simulink library "Telemaster_Lib"  (R2024b)
settings: Solver=VariableStepAuto  StartTime=0.0  StopTime=10.0  RelTol=1e-3
undefined symbols (not defined in the file): aircraft, alpha, beta, CD0, CL0, CLa, Clb, Clda, CLde, Cldr, Clp, CLq, Clr, CM0, CMa, CMde, CMq, Cnb, Cnda, Cndr, Cnp, Cnr, CYb, CYda, CYdr, CYp, CYr, dt, Earth, HM_ail, HM_ele, HM_rud, Hmalpha, Hmbeta, Hmele, Hmrud, motor, TO, WGS84
libraries: simulink_extras x21, simulink x4, aerolibtransform2 x2, shared6dof x1, aerolibatmos2 x1, aerolibasang x1, shared6dofsys x1
settings Model: Creator=igmso  LastModifiedBy=MASTER
settings RTWCC: GPUComputeCapability=3.5

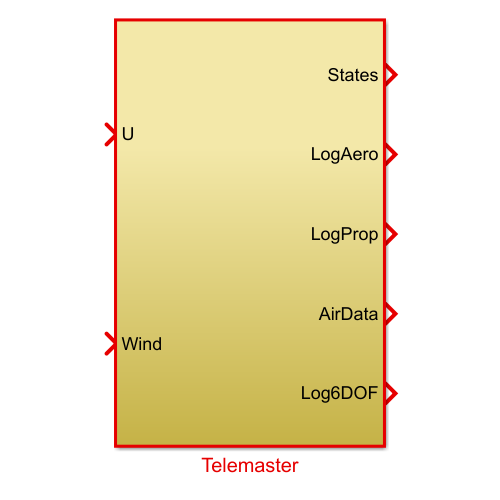
[thumbnail: Simulink's stored preview of the top-level diagram]
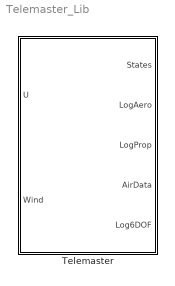
== system Telemaster_Lib ==
  Telemaster : Subsystem  TreatAsAtomicUnit=on

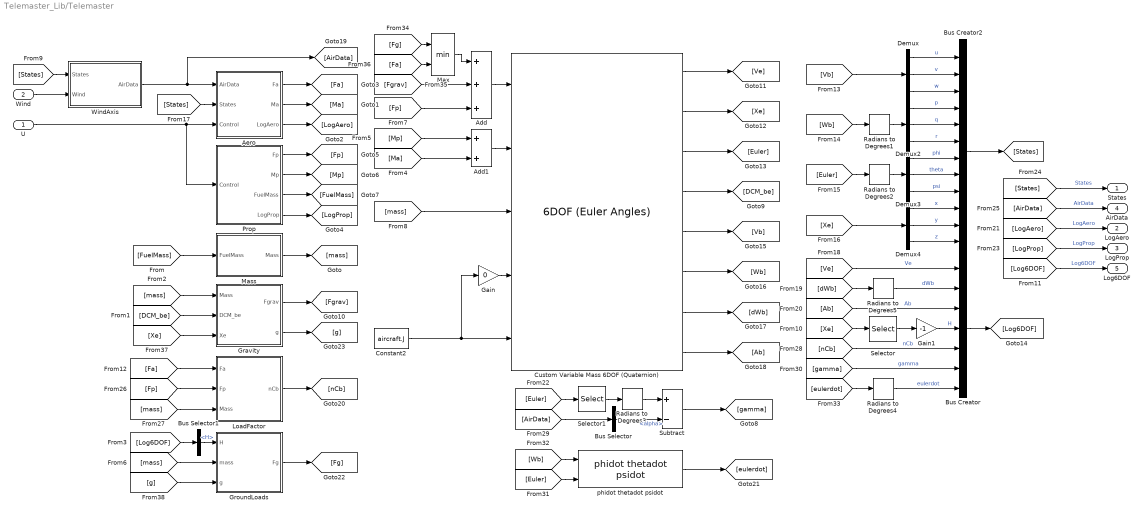
== system Telemaster_Lib/Telemaster ==
  U : Inport  SampleTime=dt
  Wind : Inport  Port=2  SampleTime=dt
  Add : Sum  Inputs=3
  Add1 : Sum
  Aero : Subsystem
  Bus Creator : BusCreator  Inputs=7
  Bus Creator2 : BusCreator  Inputs=12
  Bus Selector : BusSelector  OutputSignals=alpha
  Bus Selector1 : BusSelector  OutputSignals=H
  Constant2 : Constant  Value=aircraft.J  SampleTime=-1
  Custom Variable Mass 6DOF (Quaternion) : shared6dof/6DOF (Euler Angles)  units=Metric (MKS)  mtype=Custom Variable  rep=Euler Angles  xme_0=[TO.x TO.y TO.z-TO.alt0]  Vm_0=[TO.u TO.v TO.w]  eul_0=[TO.phi TO.theta TO.psi]  pm_0=[TO.p TO.q TO.r]  mass_0=1.0  mass_e=0.5  mass_f=2.0  inertia=eye(3)  inertia_e=eye(3)  inertia_f=2*eye(3)  k_quat=1.0  vre_flag=off  abi_flag=off  aMode=0  xme_statename={'Xe', 'Ye', 'Ze'}  Vm_statename={'u','v','w'}  eul_statename={'phi','theta','psi'}  quat_statename={'qr', 'qi', 'qj', 'qk'}  pm_statename={'p', 'q', 'r'}  mass_statename=''
  Demux{,2..4} (4 alike) : Demux  Outputs=3
  Gain : Gain  Gain=0
  Gain1 : Gain  Gain=-1
  Gravity : Subsystem
  GroundLoads : Subsystem
  LoadFactor : Subsystem
  Mass : Subsystem
  Max : MinMax  Inputs=2
  Prop : Subsystem
  Radians to Degrees{1..5} (5 alike) : simulink_extras/Transformations/Radians to Degrees
  Selector : Selector  InputPortWidth=3  IndexOptions=Index vector (dialog)  Indices=3  OutputSizes=1
  Selector1 : Selector  InputPortWidth=3  IndexOptions=Index vector (dialog)  Indices=2  OutputSizes=1
  Subtract : Sum  Inputs=+-
  WindAxis : Subsystem
  phidot thetadot psidot : shared6dofsys/DCM & Euler Angles (Euler)/phidot thetadot psidot  SystemSampleTime=-1  VariantActivationTime=update diagram  AllowFlexibleInterface=on  Latency=0  AutoFrameSizeCalculation=off
  States : Outport  SampleTime=dt
  LogAero : Outport  Port=2  SampleTime=dt
  LogProp : Outport  Port=3  SampleTime=dt
  AirData : Outport  Port=4  SampleTime=dt
  Log6DOF : Outport  Port=5  SampleTime=dt
  wires:
  [Ma] -> Add1/2
  [g] -> GroundLoads/3(g)
  Gravity/2(g) -> [g]
  [Xe] -> Gravity/3(Xe)
  [mass] -> GroundLoads/2(mass)
  Add1/1 -> Custom Variable Mass 6DOF (Quaternion)/2
  [Fa] -> Max/2
  [Fp] -> Add/3
  Max/1 -> Add/1
  [Fg] -> Max/1
  [Fgrav] -> Add/2
  Add/1 -> Custom Variable Mass 6DOF (Quaternion)/1
  [Mp] -> Add1/1
  GroundLoads/1(Fg) -> [Fg]
  Bus Selector1/1 -> GroundLoads/1(H)  "<H>"
  [Log6DOF] -> Bus Selector1/1
  Radians to Degrees5/1 -> Bus Creator/2  "dWb"
  Radians to Degrees4/1 -> Bus Creator/7  "eulerdot"
  [eulerdot] -> Radians to Degrees4/1
  phidot thetadot psidot/1 -> [eulerdot]
  [Wb] -> phidot thetadot psidot/1
  [Euler] -> phidot thetadot psidot/2
  Subtract/1 -> [gamma]
  Bus Selector/1 -> Subtract/2  "<alpha>"
  [AirData] -> Bus Selector/1
  Selector1/1 -> Radians to Degrees3/1
  Radians to Degrees3/1 -> Subtract/1
  [Euler] -> Selector1/1
  [gamma] -> Bus Creator/6  "gamma"
  [nCb] -> Bus Creator/5  "nCb"
  LoadFactor/1(nCb) -> [nCb]
  [mass] -> LoadFactor/3(Mass)
  [Fa] -> LoadFactor/1(Fa)
  [Fp] -> LoadFactor/2(Fp)
  [Log6DOF] -> Log6DOF/1  "Log6DOF"
  Bus Creator/1 -> [Log6DOF]
  Gain1/1 -> Bus Creator/4  "H"
  Selector/1 -> Gain1/1
  [Xe] -> Selector/1
  [Ab] -> Bus Creator/3  "Ab"
  [dWb] -> Radians to Degrees5/1
  [Ve] -> Bus Creator/1  "Ve"
  [States] -> States/1  "States"
  [LogProp] -> LogProp/1  "LogProp"
  [LogAero] -> LogAero/1  "LogAero"
  [AirData] -> AirData/1  "AirData"
  U/1 -> Aero/3(Control), Prop/1(Control)
  Demux3/3 -> Bus Creator2/9  "psi"
  Custom Variable Mass 6DOF (Quaternion)/4 -> [DCM_be]
  Demux3/1 -> Bus Creator2/7  "phi"
  Bus Creator2/1 -> [States]
  Custom Variable Mass 6DOF (Quaternion)/3 -> [Euler]
  Wind/1 -> WindAxis/2(Wind)
  [mass] -> Gravity/1(Mass)
  Demux4/2 -> Bus Creator2/11  "y"
  Custom Variable Mass 6DOF (Quaternion)/7 -> [dWb]
  Demux/3 -> Bus Creator2/3  "w"
  Aero/2(Ma) -> [Ma]
  Aero/1(Fa) -> [Fa]
  Custom Variable Mass 6DOF (Quaternion)/8 -> [Ab]
  [FuelMass] -> Mass/1(FuelMass)
  Demux3/2 -> Bus Creator2/8  "theta"
  Demux/2 -> Bus Creator2/2  "v"
  [States] -> Aero/2(States)
  [mass] -> Custom Variable Mass 6DOF (Quaternion)/3
  Custom Variable Mass 6DOF (Quaternion)/2 -> [Xe]
  [Vb] -> Demux/1
  Gain/1 -> Custom Variable Mass 6DOF (Quaternion)/4
  Gravity/1(Fgrav) -> [Fgrav]
  Constant2/1 -> Custom Variable Mass 6DOF (Quaternion)/5, Gain/1
  Radians to Degrees2/1 -> Demux3/1
  Mass/1(Mass) -> [mass]
  Prop/3(FuelMass) -> [FuelMass]
  Demux4/1 -> Bus Creator2/10  "x"
  Custom Variable Mass 6DOF (Quaternion)/1 -> [Ve]
  [Euler] -> Radians to Degrees2/1
  Demux2/2 -> Bus Creator2/5  "q"
  Prop/2(Mp) -> [Mp]
  Demux/1 -> Bus Creator2/1  "u"
  Prop/1(Fp) -> [Fp]
  [Wb] -> Radians to Degrees1/1
  Demux2/3 -> Bus Creator2/6  "r"
  Custom Variable Mass 6DOF (Quaternion)/6 -> [Wb]
  Demux4/3 -> Bus Creator2/12  "z"
  Custom Variable Mass 6DOF (Quaternion)/5 -> [Vb]
  [States] -> WindAxis/1(States)
  Demux2/1 -> Bus Creator2/4  "p"
  WindAxis/1(AirData) -> [AirData], Aero/1(AirData)
  Aero/3(LogAero) -> [LogAero]
  [DCM_be] -> Gravity/2(DCM_be)
  [Xe] -> Demux4/1
  Prop/4(LogProp) -> [LogProp]
  Radians to Degrees1/1 -> Demux2/1

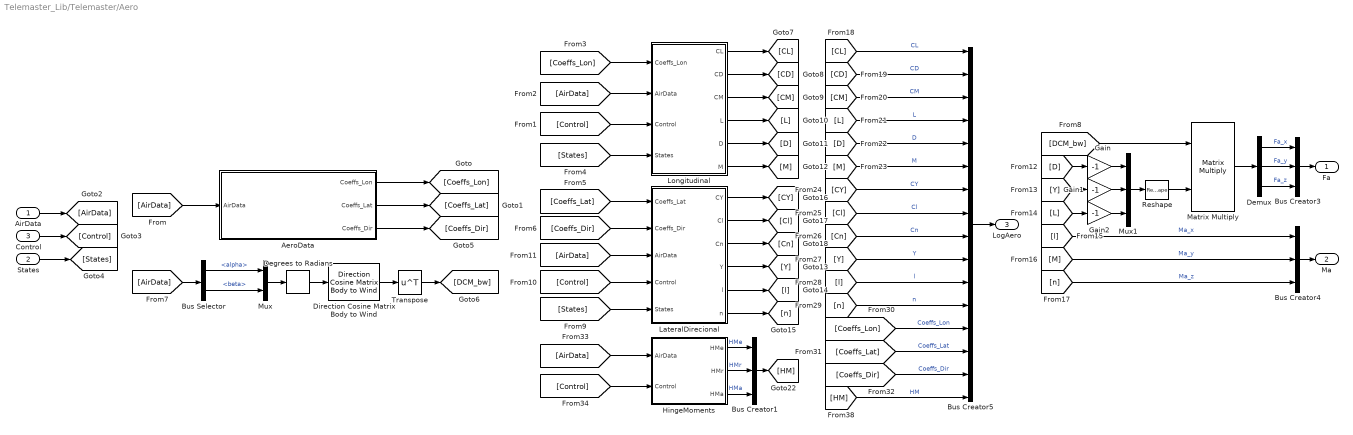
== system Telemaster_Lib/Telemaster/Aero ==
  AirData : Inport  SampleTime=dt
  States : Inport  Port=2  SampleTime=dt
  Control : Inport  Port=3  SampleTime=dt
  AeroData : Subsystem
  Bus Selector : BusSelector  OutputSignals=alpha,beta
  Bus Creator1 : BusCreator  Inputs=3
  Bus Creator3 : BusCreator  Inputs=3
  Bus Creator4 : BusCreator  Inputs=3
  Bus Creator5 : BusCreator  Inputs=16
  Degrees to Radians : simulink_extras/Transformations/Degrees to Radians
  Demux : Demux  Outputs=3
  Direction Cosine Matrix Body to Wind : aerolibtransform2/Direction Cosine Matrix Body to Wind
  Gain : Gain  Gain=-1
  Gain1 : Gain  Gain=-1
  Gain2 : Gain  Gain=-1
  HingeMoments : Subsystem
  LateralDirecional : Subsystem
  Longitudinal : Subsystem
  Matrix Multiply : Product  Multiplication=Matrix(*)
  Mux : Mux  Inputs=2
  Mux1 : Mux  Inputs=3
  Reshape : Reshape  OutputDimensionality=Column vector (2-D)
  Transpose : Math  Operator=transpose
  Fa : Outport  SampleTime=dt
  Ma : Outport  Port=2  SampleTime=dt
  LogAero : Outport  Port=3  SampleTime=dt
  wires:
  [HM] -> Bus Creator5/16  "HM"
  Reshape/1 -> Matrix Multiply/2
  Gain2/1 -> Mux1/3
  Gain1/1 -> Mux1/2
  Gain/1 -> Mux1/1
  Bus Selector/2 -> Mux/2  "<beta>"
  Bus Selector/1 -> Mux/1  "<alpha>"
  [AirData] -> Bus Selector/1
  [AirData] -> AeroData/1(AirData)
  AirData/1 -> [AirData]
  Bus Creator1/1 -> [HM]
  HingeMoments/1(HMe) -> Bus Creator1/1  "HMe"
  HingeMoments/2(HMr) -> Bus Creator1/2  "HMr"
  HingeMoments/3(HMa) -> Bus Creator1/3  "HMa"
  [Control] -> HingeMoments/2(Control)
  [AirData] -> HingeMoments/1(AirData)
  Control/1 -> [Control]
  Bus Creator4/1 -> Ma/1
  LateralDirecional/4(Y) -> [Y]
  [Coeffs_Dir] -> Bus Creator5/15  "Coeffs_Dir"
  LateralDirecional/1(CY) -> [CY]
  [L] -> Gain2/1
  Longitudinal/3(CM) -> [CM]
  [DCM_bw] -> Matrix Multiply/1
  Direction Cosine Matrix Body to Wind/1 -> Transpose/1
  [AirData] -> Longitudinal/2(AirData)
  States/1 -> [States]
  Mux1/1 -> Reshape/1
  Mux/1 -> Degrees to Radians/1
  AeroData/2(Coeffs_Lat) -> [Coeffs_Lat]
  AeroData/3(Coeffs_Dir) -> [Coeffs_Dir]
  [States] -> LateralDirecional/5(States)
  Bus Creator5/1 -> LogAero/1
  [Control] -> LateralDirecional/4(Control)
  [CL] -> Bus Creator5/1  "CL"
  Longitudinal/4(L) -> [L]
  [Coeffs_Lon] -> Bus Creator5/13  "Coeffs_Lon"
  [l] -> Bus Creator5/11  "l"
  [n] -> Bus Creator5/12  "n"
  [Cn] -> Bus Creator5/9  "Cn"
  Matrix Multiply/1 -> Demux/1
  [M] -> Bus Creator5/6  "M"
  [CM] -> Bus Creator5/3  "CM"
  Transpose/1 -> [DCM_bw]
  Longitudinal/2(CD) -> [CD]
  Bus Creator3/1 -> Fa/1
  [Coeffs_Dir] -> LateralDirecional/2(Coeffs_Dir)
  [CY] -> Bus Creator5/7  "CY"
  [M] -> Bus Creator4/2  "Ma_y"
  [D] -> Bus Creator5/5  "D"
  Longitudinal/1(CL) -> [CL]
  [L] -> Bus Creator5/4  "L"
  [l] -> Bus Creator4/1  "Ma_x"
  [Control] -> Longitudinal/3(Control)
  LateralDirecional/6(n) -> [n]
  Demux/3 -> Bus Creator3/3  "Fa_z"
  LateralDirecional/3(Cn) -> [Cn]
  LateralDirecional/5(l) -> [l]
  [Coeffs_Lat] -> LateralDirecional/1(Coeffs_Lat)
  [States] -> Longitudinal/4(States)
  Degrees to Radians/1 -> Direction Cosine Matrix Body to Wind/1
  [Y] -> Gain1/1
  Demux/1 -> Bus Creator3/1  "Fa_x"
  AeroData/1(Coeffs_Lon) -> [Coeffs_Lon]
  Demux/2 -> Bus Creator3/2  "Fa_y"
  LateralDirecional/2(Cl) -> [Cl]
  [D] -> Gain/1
  Longitudinal/5(D) -> [D]
  [Cl] -> Bus Creator5/8  "Cl"
  [Coeffs_Lat] -> Bus Creator5/14  "Coeffs_Lat"
  [n] -> Bus Creator4/3  "Ma_z"
  Longitudinal/6(M) -> [M]
  [CD] -> Bus Creator5/2  "CD"
  [Y] -> Bus Creator5/10  "Y"
  [Coeffs_Lon] -> Longitudinal/1(Coeffs_Lon)
  [AirData] -> LateralDirecional/3(AirData)

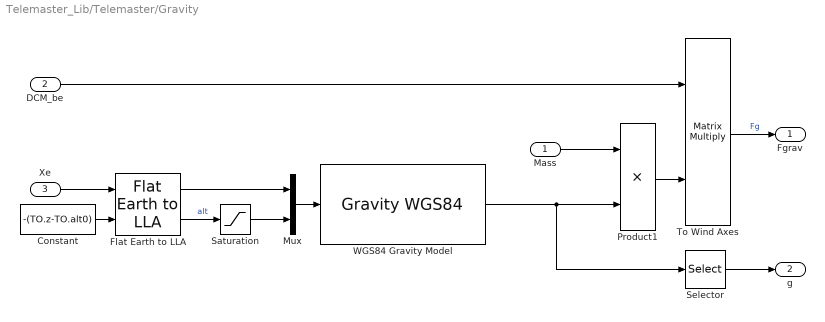
== system Telemaster_Lib/Telemaster/Gravity ==
  Mass : Inport  SampleTime=dt
  DCM_be : Inport  Port=2  SampleTime=dt
  Xe : Inport  Port=3
  Constant : Constant  Value=-(TO.z-TO.alt0)  SampleTime=-1
  Flat Earth to LLA : aerolibtransform2/Flat Earth to LLA  units=Metric (MKS)  ptype=Earth (WGS84)  F=1/298.257223563  R=6378137  refPosPort=off  LL0=[-23.2296 -45.8614].'  psi=150
  Mux : Mux  Inputs=2
  Product1 : Product
  Saturation : Saturate  UpperLimit=20e3  LowerLimit=0
  Selector : Selector  InputPortWidth=3  IndexOptions=Index vector (dialog)  Indices=3  OutputSizes=1
  To Wind Axes : Product  Multiplication=Matrix(*)  InputSameDT=on  SaturateOnIntegerOverflow=on  OutDataTypeStr=Inherit: Same as first input
  "WGS84 Gravity Model  " : GravityWGS84
  Fgrav : Outport  SampleTime=dt
  g : Outport  Port=2
  wires:
  Selector/1 -> g/1
  Mass/1 -> Product1/1
  Saturation/1 -> Mux/2
  Xe/1 -> Flat Earth to LLA/1
  "WGS84 Gravity Model  "/1 -> Product1/2, Selector/1
  Flat Earth to LLA/1 -> Mux/1
  DCM_be/1 -> To Wind Axes/1
  To Wind Axes/1 -> Fgrav/1  "Fg"
  Product1/1 -> To Wind Axes/2
  Mux/1 -> "WGS84 Gravity Model  "/1
  Flat Earth to LLA/2 -> Saturation/1  "alt"
  Constant/1 -> Flat Earth to LLA/2

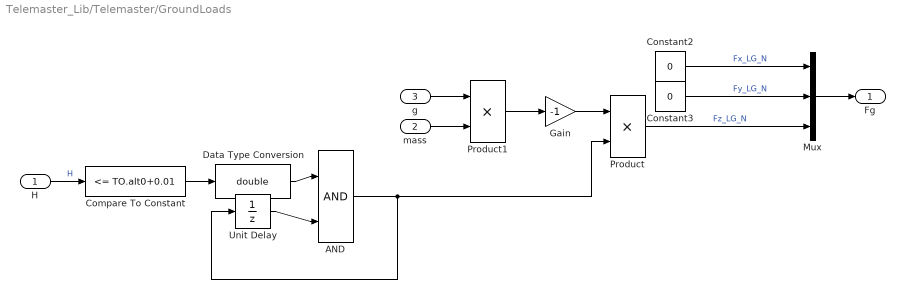
== system Telemaster_Lib/Telemaster/GroundLoads ==
  H : Inport
  mass : Inport  Port=2
  g : Inport  Port=3
  AND : Logic  IconShape=distinctive  AllPortsSameDT=off  OutDataTypeStr=boolean
  Compare To Constant : simulink/Logic and Bit Operations/Compare To Constant  relop=<=  const=TO.alt0+0.01  OutDataTypeStr=boolean
  Constant2 : Constant  Value=0  SampleTime=-1
  Constant3 : Constant  Value=0  SampleTime=-1
  Data Type Conversion : DataTypeConversion  OutDataTypeStr=double  SaturateOnIntegerOverflow=off  RndMeth=Floor
  Gain : Gain  Gain=-1
  Mux : Mux  Inputs=3
  Product : Product
  Product1 : Product
  Unit Delay : UnitDelay  InitialCondition=1  SampleTime=-1  HasFrameUpgradeWarning=on
  Fg : Outport
  wires:
  AND/1 -> Unit Delay/1, Product/2
  Gain/1 -> Product/1
  g/1 -> Product1/1
  Mux/1 -> Fg/1
  Product/1 -> Mux/3  "Fz_LG_N"
  Constant3/1 -> Mux/2  "Fy_LG_N"
  Constant2/1 -> Mux/1  "Fx_LG_N"
  H/1 -> Compare To Constant/1  "H"
  Compare To Constant/1 -> Data Type Conversion/1
  Product1/1 -> Gain/1
  mass/1 -> Product1/2
  Data Type Conversion/1 -> AND/1
  Unit Delay/1 -> AND/2

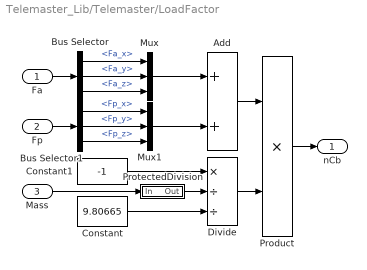
== system Telemaster_Lib/Telemaster/LoadFactor ==
  Fa : Inport  SampleTime=dt
  Fp : Inport  Port=2  SampleTime=dt
  Mass : Inport  Port=3  SampleTime=dt
  Add : Sum  Inputs=2
  Bus Selector : BusSelector  OutputSignals=Fa_x,Fa_y,Fa_z
  Bus Selector1 : BusSelector  OutputSignals=Fp_x,Fp_y,Fp_z
  Constant : Constant  Value=9.80665  SampleTime=dt
  Constant1 : Constant  Value=-1  SampleTime=dt
  Divide : Product  Inputs=*//
  Mux : Mux  Inputs=3
  Mux1 : Mux  Inputs=3
  Product : Product
  ProtectedDivision : Subsystem
  nCb : Outport  SampleTime=dt
  wires:
  ProtectedDivision/1(Out) -> Divide/2
  Product/1 -> nCb/1
  Divide/1 -> Product/2
  Constant/1 -> Divide/3
  Mass/1 -> ProtectedDivision/1(In)
  Constant1/1 -> Divide/1
  Add/1 -> Product/1
  Fa/1 -> Bus Selector/1
  Bus Selector/1 -> Mux/1  "<Fa_x>"
  Bus Selector/2 -> Mux/2  "<Fa_y>"
  Bus Selector/3 -> Mux/3  "<Fa_z>"
  Fp/1 -> Bus Selector1/1
  Bus Selector1/1 -> Mux1/1  "<Fp_x>"
  Bus Selector1/2 -> Mux1/2  "<Fp_y>"
  Bus Selector1/3 -> Mux1/3  "<Fp_z>"
  Mux/1 -> Add/1
  Mux1/1 -> Add/2

== system Telemaster_Lib/Telemaster/Mass ==
  FuelMass : Inport  SampleTime=dt
  Add : Sum
  Constant1 : Constant  Value=aircraft.m  SampleTime=dt
  Mass : Outport  SampleTime=dt
  wires:
  Add/1 -> Mass/1
  FuelMass/1 -> Add/2
  Constant1/1 -> Add/1

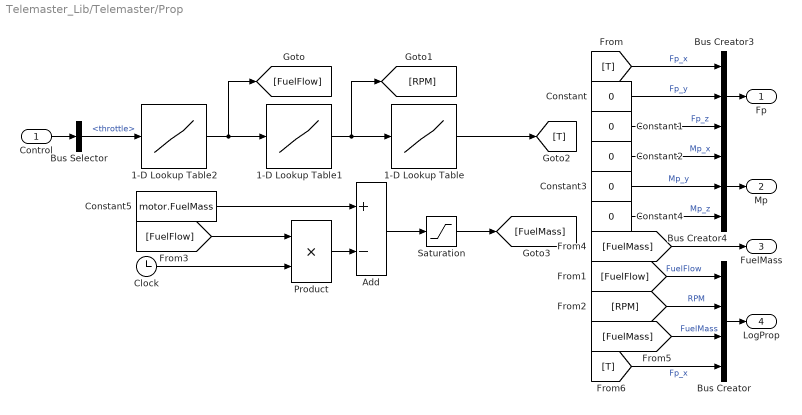
== system Telemaster_Lib/Telemaster/Prop ==
  Control : Inport  SampleTime=dt
  1-D Lookup Table : Lookup_n-D  NumberOfTableDimensions=1  BreakpointsForDimension1=[1600 6600]  Table=[0 28.4]  ExtrapMethod=Clip  InternalRulePriority=Speed  RndMeth=Simplest
  1-D Lookup Table1 : Lookup_n-D  NumberOfTableDimensions=1  BreakpointsForDimension1=[0.0002 0.001]  Table=[1600 6600]  ExtrapMethod=Clip  InternalRulePriority=Speed  RndMeth=Simplest
  1-D Lookup Table2 : Lookup_n-D  NumberOfTableDimensions=1  BreakpointsForDimension1=[0 1]  Table=[0.0002 0.001]  ExtrapMethod=Clip  InternalRulePriority=Speed  RndMeth=Simplest
  Add : Sum  Inputs=+-
  Bus Selector : BusSelector  OutputSignals=throttle
  Bus Creator : BusCreator  Inputs=4
  Bus Creator3 : BusCreator  Inputs=3
  Bus Creator4 : BusCreator  Inputs=3
  Clock : Clock
  Constant{,1..4} (5 alike) : Constant  Value=0  SampleTime=-1
  Constant5 : Constant  Value=motor.FuelMass  SampleTime=-1
  Product : Product
  Saturation : Saturate  UpperLimit=inf  LowerLimit=0
  Fp : Outport  SampleTime=dt
  Mp : Outport  Port=2  SampleTime=dt
  FuelMass : Outport  Port=3  SampleTime=dt
  LogProp : Outport  Port=4  SampleTime=dt
  wires:
  [T] -> Bus Creator/4  "Fp_x"
  Clock/1 -> Product/2
  1-D Lookup Table2/1 -> 1-D Lookup Table1/1, [FuelFlow]
  1-D Lookup Table1/1 -> 1-D Lookup Table/1, [RPM]
  1-D Lookup Table/1 -> [T]
  Bus Selector/1 -> 1-D Lookup Table2/1  "<throttle>"
  [FuelMass] -> Bus Creator/3  "FuelMass"
  [FuelFlow] -> Bus Creator/1  "FuelFlow"
  Saturation/1 -> [FuelMass]
  Bus Creator/1 -> LogProp/1
  [RPM] -> Bus Creator/2  "RPM"
  [FuelMass] -> FuelMass/1
  Add/1 -> Saturation/1
  Product/1 -> Add/2
  [FuelFlow] -> Product/1
  Constant5/1 -> Add/1
  Constant2/1 -> Bus Creator4/1  "Mp_x"
  Constant3/1 -> Bus Creator4/2  "Mp_y"
  [T] -> Bus Creator3/1  "Fp_x"
  Control/1 -> Bus Selector/1
  Constant/1 -> Bus Creator3/2  "Fp_y"
  Constant1/1 -> Bus Creator3/3  "Fp_z"
  Bus Creator3/1 -> Fp/1
  Bus Creator4/1 -> Mp/1
  Constant4/1 -> Bus Creator4/3  "Mp_z"

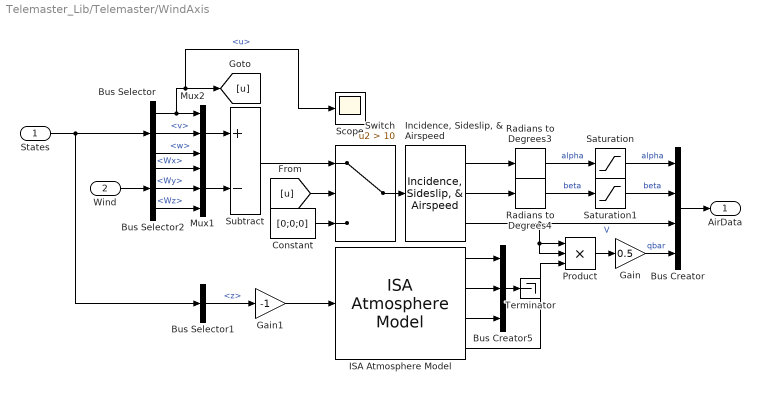
== system Telemaster_Lib/Telemaster/WindAxis ==
  States : Inport  SampleTime=dt
  Wind : Inport  Port=2  SampleTime=dt
  Bus Selector : BusSelector  OutputSignals=u,v,w
  Bus Selector1 : BusSelector  OutputSignals=z
  Bus Selector2 : BusSelector  OutputSignals=Wx,Wy,Wz
  Bus Creator : BusCreator  Inputs=4
  Bus Creator5 : BusCreator  Inputs=3
  Constant : Constant  Value=[0;0;0]  SampleTime=-1
  Gain : Gain  Gain=0.5
  Gain1 : Gain  Gain=-1
  ISA Atmosphere Model : aerolibatmos2/ISA Atmosphere Model  useExtended=off  action=Warning  custom=off  viscosityOut=off  g=9.80665  gamma=1.4  R=287.0531  L=0.0065  h_trop=11000  h_strat=20000  rho0=1.225  P0=101325  T0=288.15  h0=0  S=110.4  Tref=273.15  muref=1.716e-5
  "Incidence, Sideslip, & Airspeed" : aerolibasang/Incidence, Sideslip, & Airspeed
  Mux1 : Mux  Inputs=3
  Mux2 : Mux  Inputs=3
  Product : Product  Inputs=3
  Radians to Degrees3 : simulink_extras/Transformations/Radians to Degrees
  Radians to Degrees4 : simulink_extras/Transformations/Radians to Degrees
  Saturation : Saturate  UpperLimit=15  LowerLimit=-10
  Saturation1 : Saturate  UpperLimit=10  LowerLimit=-10
  Scope : Scope
  Subtract : Sum  Inputs=+-
  Switch : Switch  Criteria=u2 > Threshold  Threshold=10  SaturateOnIntegerOverflow=off  InputSameDT=off
  Terminator : Terminator
  AirData : Outport  SampleTime=dt
  wires:
  Constant/1 -> Switch/3
  Switch/1 -> "Incidence, Sideslip, & Airspeed"/1
  [u] -> Switch/2
  Saturation1/1 -> Bus Creator/2  "beta"
  Saturation/1 -> Bus Creator/1  "alpha"
  Mux2/1 -> Subtract/1
  Product/1 -> Gain/1
  Wind/1 -> Bus Selector2/1
  Bus Selector2/3 -> Mux1/3  "<Wz>"
  Bus Selector2/1 -> Mux1/1  "<Wx>"
  Mux1/1 -> Subtract/2
  Bus Selector2/2 -> Mux1/2  "<Wy>"
  Bus Creator/1 -> AirData/1
  "Incidence, Sideslip, & Airspeed"/1 -> Radians to Degrees3/1
  ISA Atmosphere Model/2 -> Bus Creator5/2
  ISA Atmosphere Model/1 -> Bus Creator5/1
  Radians to Degrees4/1 -> Saturation1/1  "beta"
  Gain/1 -> Bus Creator/4  "qbar"
  Bus Selector/2 -> Mux2/2  "<v>"
  ISA Atmosphere Model/4 -> Product/3
  ISA Atmosphere Model/3 -> Bus Creator5/3
  Bus Selector/1 -> Mux2/1, [u], Scope/1  "<u>"
  Radians to Degrees3/1 -> Saturation/1  "alpha"
  Bus Selector1/1 -> Gain1/1  "<z>"
  Gain1/1 -> ISA Atmosphere Model/1
  "Incidence, Sideslip, & Airspeed"/3 -> Product/1, Product/2, Bus Creator/3  "V"
  States/1 -> Bus Selector/1, Bus Selector1/1
  Bus Creator5/1 -> Terminator/1
  "Incidence, Sideslip, & Airspeed"/2 -> Radians to Degrees4/1
  Subtract/1 -> Switch/1
  Bus Selector/3 -> Mux2/3  "<w>"

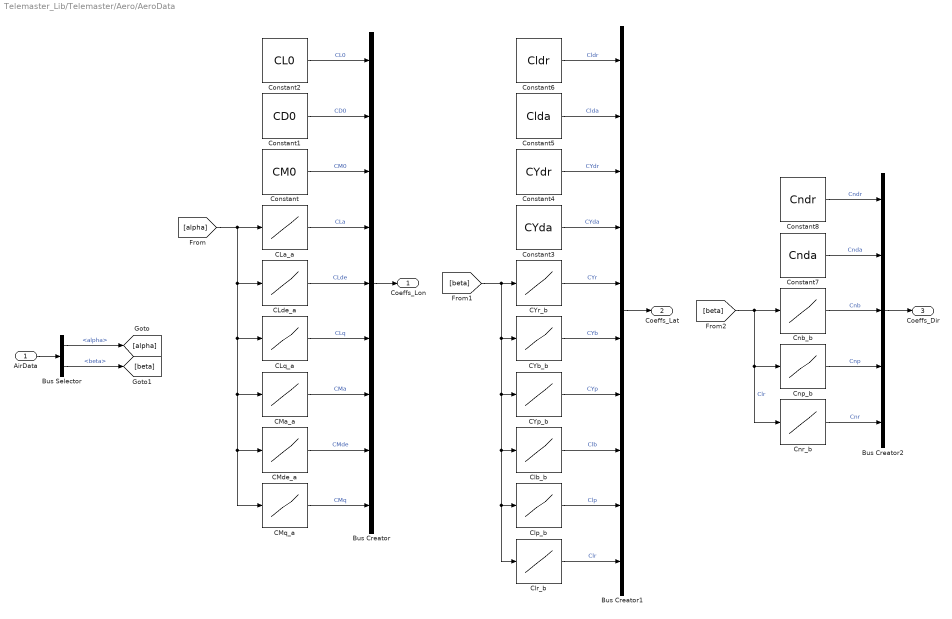
== system Telemaster_Lib/Telemaster/Aero/AeroData ==
  AirData : Inport
  Bus Selector : BusSelector  OutputSignals=alpha,beta
  Bus Creator : BusCreator  Inputs=9
  Bus Creator1 : BusCreator  Inputs=10
  Bus Creator2 : BusCreator  Inputs=5
  CLa_a : Lookup_n-D  NumberOfTableDimensions=1  BreakpointsForDimension1=alpha  Table=CLa  InternalRulePriority=Speed  RndMeth=Simplest
  CLde_a : Lookup_n-D  NumberOfTableDimensions=1  BreakpointsForDimension1=alpha  Table=CLde  InternalRulePriority=Speed  RndMeth=Simplest
  CLq_a : Lookup_n-D  NumberOfTableDimensions=1  BreakpointsForDimension1=alpha  Table=CLq  InternalRulePriority=Speed  RndMeth=Simplest
  CMa_a : Lookup_n-D  NumberOfTableDimensions=1  BreakpointsForDimension1=alpha  Table=CMa  InternalRulePriority=Speed  RndMeth=Simplest
  CMde_a : Lookup_n-D  NumberOfTableDimensions=1  BreakpointsForDimension1=alpha  Table=CMde  InternalRulePriority=Speed  RndMeth=Simplest
  CMq_a : Lookup_n-D  NumberOfTableDimensions=1  BreakpointsForDimension1=alpha  Table=CMq  InternalRulePriority=Speed  RndMeth=Simplest
  CYb_b : Lookup_n-D  NumberOfTableDimensions=1  BreakpointsForDimension1=beta  Table=CYb  InternalRulePriority=Speed  RndMeth=Simplest
  CYp_b : Lookup_n-D  NumberOfTableDimensions=1  BreakpointsForDimension1=beta  Table=CYp  InternalRulePriority=Speed  RndMeth=Simplest
  CYr_b : Lookup_n-D  NumberOfTableDimensions=1  BreakpointsForDimension1=beta  Table=CYr  InternalRulePriority=Speed  RndMeth=Simplest
  Clb_b : Lookup_n-D  NumberOfTableDimensions=1  BreakpointsForDimension1=beta  Table=Clb  InternalRulePriority=Speed  RndMeth=Simplest
  Clp_b : Lookup_n-D  NumberOfTableDimensions=1  BreakpointsForDimension1=beta  Table=Clp  InternalRulePriority=Speed  RndMeth=Simplest
  Clr_b : Lookup_n-D  NumberOfTableDimensions=1  BreakpointsForDimension1=beta  Table=Clr  InternalRulePriority=Speed  RndMeth=Simplest
  Cnb_b : Lookup_n-D  NumberOfTableDimensions=1  BreakpointsForDimension1=beta  Table=Cnb  InternalRulePriority=Speed  RndMeth=Simplest
  Cnp_b : Lookup_n-D  NumberOfTableDimensions=1  BreakpointsForDimension1=beta  Table=Cnp  InternalRulePriority=Speed  RndMeth=Simplest
  Cnr_b : Lookup_n-D  NumberOfTableDimensions=1  BreakpointsForDimension1=beta  Table=Cnr  InternalRulePriority=Speed  RndMeth=Simplest
  Constant : Constant  Value=CM0  SampleTime=-1
  Constant1 : Constant  Value=CD0  SampleTime=-1
  Constant2 : Constant  Value=CL0  SampleTime=-1
  Constant3 : Constant  Value=CYda  SampleTime=-1
  Constant4 : Constant  Value=CYdr  SampleTime=-1
  Constant5 : Constant  Value=Clda  SampleTime=-1
  Constant6 : Constant  Value=Cldr  SampleTime=-1
  Constant7 : Constant  Value=Cnda  SampleTime=-1
  Constant8 : Constant  Value=Cndr  SampleTime=-1
  Coeffs_Lon : Outport
  Coeffs_Lat : Outport  Port=2
  Coeffs_Dir : Outport  Port=3
  wires:
  Bus Selector/2 -> [beta]  "<beta>"
  Bus Selector/1 -> [alpha]  "<alpha>"
  AirData/1 -> Bus Selector/1
  Clr_b/1 -> Bus Creator1/10  "Clr"
  CYr_b/1 -> Bus Creator1/5  "CYr"
  Bus Creator2/1 -> Coeffs_Dir/1
  Cnp_b/1 -> Bus Creator2/4  "Cnp"
  Cnr_b/1 -> Bus Creator2/5  "Cnr"
  Cnb_b/1 -> Bus Creator2/3  "Cnb"
  [beta] -> Cnb_b/1, Cnp_b/1, Cnr_b/1  "Clr"
  Constant7/1 -> Bus Creator2/2  "Cnda"
  Constant8/1 -> Bus Creator2/1  "Cndr"
  Constant6/1 -> Bus Creator1/1  "Cldr"
  Constant5/1 -> Bus Creator1/2  "Clda"
  Constant4/1 -> Bus Creator1/3  "CYdr"
  Constant3/1 -> Bus Creator1/4  "CYda"
  Constant2/1 -> Bus Creator/1  "CL0"
  Constant1/1 -> Bus Creator/2  "CD0"
  Constant/1 -> Bus Creator/3  "CM0"
  Bus Creator1/1 -> Coeffs_Lat/1
  Bus Creator/1 -> Coeffs_Lon/1
  CLa_a/1 -> Bus Creator/4  "CLa"
  CMa_a/1 -> Bus Creator/7  "CMa"
  Clp_b/1 -> Bus Creator1/9  "Clp"
  CLde_a/1 -> Bus Creator/5  "CLde"
  CYb_b/1 -> Bus Creator1/6  "CYb"
  CMq_a/1 -> Bus Creator/9  "CMq"
  CLq_a/1 -> Bus Creator/6  "CLq"
  CYp_b/1 -> Bus Creator1/7  "CYp"
  Clb_b/1 -> Bus Creator1/8  "Clb"
  [beta] -> CYb_b/1, CYp_b/1, Clb_b/1, Clp_b/1, Clr_b/1, CYr_b/1
  CMde_a/1 -> Bus Creator/8  "CMde"
  [alpha] -> CLa_a/1, CLde_a/1, CLq_a/1, CMa_a/1, CMde_a/1, CMq_a/1

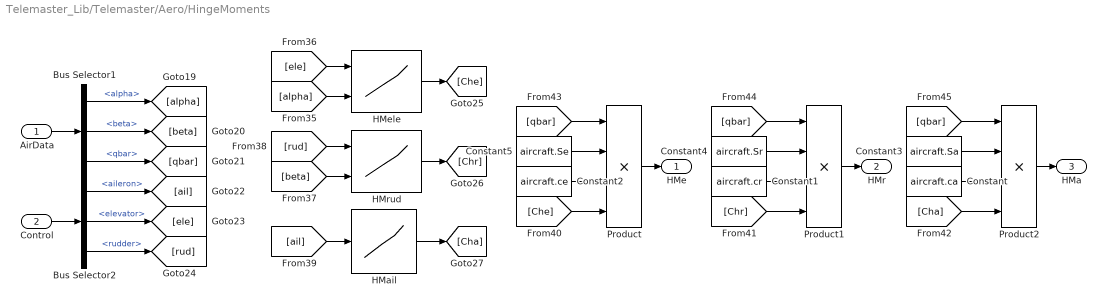
== system Telemaster_Lib/Telemaster/Aero/HingeMoments ==
  AirData : Inport
  Control : Inport  Port=2
  Bus Selector1 : BusSelector  OutputSignals=alpha,beta,qbar
  Bus Selector2 : BusSelector  OutputSignals=aileron,elevator,rudder
  Constant : Constant  Value=aircraft.ca  SampleTime=-1
  Constant1 : Constant  Value=aircraft.cr  SampleTime=-1
  Constant2 : Constant  Value=aircraft.ce  SampleTime=-1
  Constant3 : Constant  Value=aircraft.Sa  SampleTime=-1
  Constant4 : Constant  Value=aircraft.Sr  SampleTime=-1
  Constant5 : Constant  Value=aircraft.Se  SampleTime=-1
  HMail : Lookup_n-D  NumberOfTableDimensions=1  BreakpointsForDimension1=Hmrud  Table=HM_ail  InternalRulePriority=Speed  RndMeth=Simplest
  HMele : Lookup_n-D  BreakpointsForDimension1=Hmele  BreakpointsForDimension2=Hmalpha  Table=HM_ele  InternalRulePriority=Speed  RndMeth=Simplest
      settings: InputPortMap=u0,u1
  HMrud : Lookup_n-D  BreakpointsForDimension1=Hmrud  BreakpointsForDimension2=Hmbeta  Table=HM_rud  InternalRulePriority=Speed  RndMeth=Simplest
      settings: InputPortMap=u0,u1
  Product : Product  Inputs=4
  Product1 : Product  Inputs=4
  Product2 : Product  Inputs=4
  HMe : Outport
  HMr : Outport  Port=2
  HMa : Outport  Port=3
  wires:
  Product1/1 -> HMr/1
  Control/1 -> Bus Selector2/1
  AirData/1 -> Bus Selector1/1
  Bus Selector2/3 -> [rud]  "<rudder>"
  Bus Selector2/1 -> [ail]  "<aileron>"
  Constant4/1 -> Product1/2
  HMele/1 -> [Che]
  [rud] -> HMrud/1
  HMrud/1 -> [Chr]
  [ele] -> HMele/1
  [qbar] -> Product/1
  Bus Selector1/3 -> [qbar]  "<qbar>"
  Constant5/1 -> Product/2
  Constant2/1 -> Product/3
  Constant1/1 -> Product1/3
  [Chr] -> Product1/4
  Product2/1 -> HMa/1
  [Che] -> Product/4
  [beta] -> HMrud/2
  [qbar] -> Product1/1
  Bus Selector1/1 -> [alpha]  "<alpha>"
  Product/1 -> HMe/1
  [alpha] -> HMele/2
  Constant/1 -> Product2/3
  [qbar] -> Product2/1
  [Cha] -> Product2/4
  [ail] -> HMail/1
  Bus Selector1/2 -> [beta]  "<beta>"
  Constant3/1 -> Product2/2
  Bus Selector2/2 -> [ele]  "<elevator>"
  HMail/1 -> [Cha]

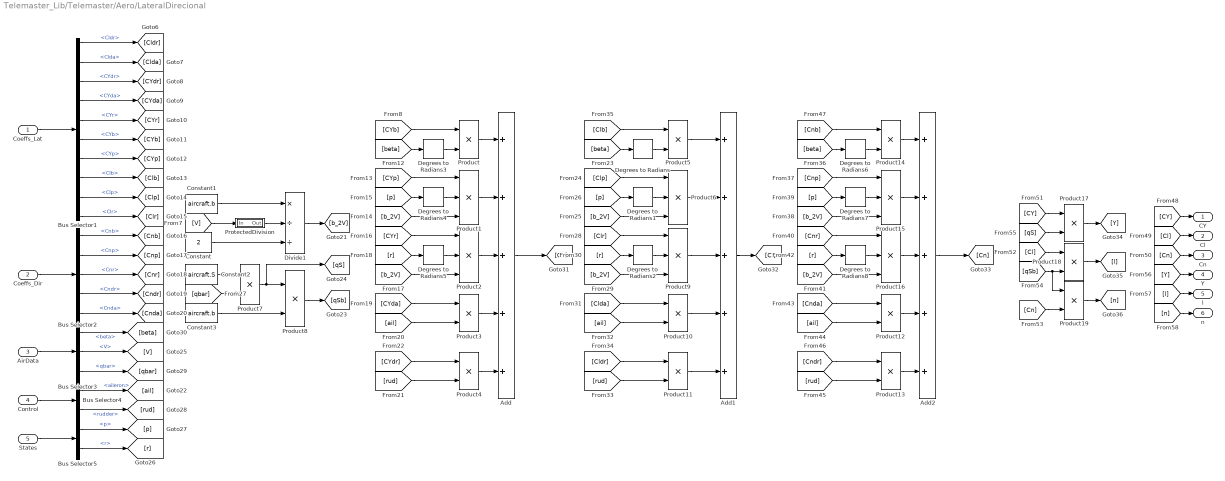
== system Telemaster_Lib/Telemaster/Aero/LateralDirecional ==
  Coeffs_Lat : Inport
  Coeffs_Dir : Inport  Port=2
  AirData : Inport  Port=3
  Control : Inport  Port=4
  States : Inport  Port=5
  Add : Sum  Inputs=5
  Add1 : Sum  Inputs=5
  Add2 : Sum  Inputs=5
  Bus Selector1 : BusSelector  OutputSignals=Cldr,Clda,CYdr,CYda,CYr,CYb,CYp,Clb,Clp,Clr
  Bus Selector2 : BusSelector  OutputSignals=Cnb,Cnp,Cnr,Cndr,Cnda
  Bus Selector3 : BusSelector  OutputSignals=beta,V,qbar
  Bus Selector4 : BusSelector  OutputSignals=aileron,rudder
  Bus Selector5 : BusSelector  OutputSignals=p,r
  Constant : Constant  Value=2  SampleTime=-1
  Constant1 : Constant  Value=aircraft.b  SampleTime=-1
  Constant2 : Constant  Value=aircraft.S
  Constant3 : Constant  Value=aircraft.b
  Degrees to Radians{,1..8} (9 alike) : simulink_extras/Transformations/Degrees to Radians
  Divide1 : Product  Inputs=*//
  Product{,3..5,7..8,10..14,17..19} (14 alike) : Product
  Product{1..2,6,9,15..16} (6 alike) : Product  Inputs=3
  ProtectedDivision : Subsystem
  CY : Outport
  Cl : Outport  Port=2
  Cn : Outport  Port=3
  Y : Outport  Port=4
  l : Outport  Port=5
  n : Outport  Port=6
  wires:
  ProtectedDivision/1(Out) -> Divide1/2
  [n] -> n/1
  Coeffs_Dir/1 -> Bus Selector2/1
  [Cl] -> Cl/1
  [CY] -> CY/1
  [l] -> l/1
  Control/1 -> Bus Selector4/1
  States/1 -> Bus Selector5/1
  Coeffs_Lat/1 -> Bus Selector1/1
  AirData/1 -> Bus Selector3/1
  Degrees to Radians/1 -> Product5/2
  Degrees to Radians2/1 -> Product9/2
  Product17/1 -> [Y]
  Add/1 -> [CY]
  [CYb] -> Product/1
  Bus Selector1/10 -> [Clr]  "<Clr>"
  [Clp] -> Product6/1
  [p] -> Degrees to Radians1/1
  [b_2V] -> Product6/3
  [Clb] -> Product5/1
  [Clda] -> Product10/1
  Product9/1 -> Add1/3
  Product5/1 -> Add1/1
  [ail] -> Product10/2
  [Clr] -> Product9/1
  Product10/1 -> Add1/4
  [r] -> Degrees to Radians2/1
  [b_2V] -> Product9/3
  Product6/1 -> Add1/2
  Add1/1 -> [Cl]
  Bus Selector2/4 -> [Cndr]  "<Cndr>"
  Bus Selector2/3 -> [Cnr]  "<Cnr>"
  Bus Selector5/1 -> [p]  "<p>"
  Degrees to Radians3/1 -> Product/2
  Bus Selector3/2 -> [V]  "<V>"
  Bus Selector4/1 -> [ail]  "<aileron>"
  Bus Selector4/2 -> [rud]  "<rudder>"
  Product19/1 -> [n]
  [p] -> Degrees to Radians4/1
  [r] -> Degrees to Radians5/1
  [b_2V] -> Product2/3
  Degrees to Radians8/1 -> Product16/2
  [CYda] -> Product3/1
  [CYdr] -> Product4/1
  Bus Selector2/1 -> [Cnb]  "<Cnb>"
  [Cldr] -> Product11/1
  [beta] -> Degrees to Radians3/1
  Bus Selector1/8 -> [Clb]  "<Clb>"
  [rud] -> Product11/2
  Degrees to Radians5/1 -> Product2/2
  Product/1 -> Add/1
  Product2/1 -> Add/3
  Divide1/1 -> [b_2V]
  [Cn] -> Product19/2
  [qbar] -> Product7/2
  [rud] -> Product4/2
  [Cl] -> Product18/1
  Degrees to Radians7/1 -> Product15/2
  Bus Selector5/2 -> [r]  "<r>"
  Product14/1 -> Add2/1
  [V] -> ProtectedDivision/1(In)
  [Cnb] -> Product14/1
  [b_2V] -> Product1/3
  Product11/1 -> Add1/5
  [ail] -> Product3/2
  Bus Selector1/9 -> [Clp]  "<Clp>"
  Bus Selector3/1 -> [beta]  "<beta>"
  Constant3/1 -> Product8/2
  Bus Selector1/7 -> [CYp]  "<CYp>"
  [Cn] -> Cn/1
  Product13/1 -> Add2/5
  [rud] -> Product13/2
  Bus Selector1/5 -> [CYr]  "<CYr>"
  [Cndr] -> Product13/1
  [qSb] -> Product18/2, Product19/1
  Bus Selector2/2 -> [Cnp]  "<Cnp>"
  Product3/1 -> Add/4
  Product15/1 -> Add2/2
  [Y] -> Y/1
  Bus Selector3/3 -> [qbar]  "<qbar>"
  [CYp] -> Product1/1
  Product16/1 -> Add2/3
  [ail] -> Product12/2
  Bus Selector2/5 -> [Cnda]  "<Cnda>"
  Bus Selector1/2 -> [Clda]  "<Clda>"
  Product7/1 -> Product8/1, [qS]
  Degrees to Radians4/1 -> Product1/2
  [Cnr] -> Product16/1
  [CYr] -> Product2/1
  [p] -> Degrees to Radians7/1
  Degrees to Radians6/1 -> Product14/2
  Bus Selector1/4 -> [CYda]  "<CYda>"
  Add2/1 -> [Cn]
  [r] -> Degrees to Radians8/1
  Bus Selector1/3 -> [CYdr]  "<CYdr>"
  Bus Selector1/1 -> [Cldr]  "<Cldr>"
  [b_2V] -> Product16/3
  [Cnda] -> Product12/1
  [qS] -> Product17/2
  [Cnp] -> Product15/1
  Product4/1 -> Add/5
  Constant/1 -> Divide1/3
  [CY] -> Product17/1
  Constant2/1 -> Product7/1
  [b_2V] -> Product15/3
  [beta] -> Degrees to Radians/1
  Constant1/1 -> Divide1/1
  Product18/1 -> [l]
  Product1/1 -> Add/2
  Bus Selector1/6 -> [CYb]  "<CYb>"
  Product12/1 -> Add2/4
  Degrees to Radians1/1 -> Product6/2
  [beta] -> Degrees to Radians6/1
  Product8/1 -> [qSb]

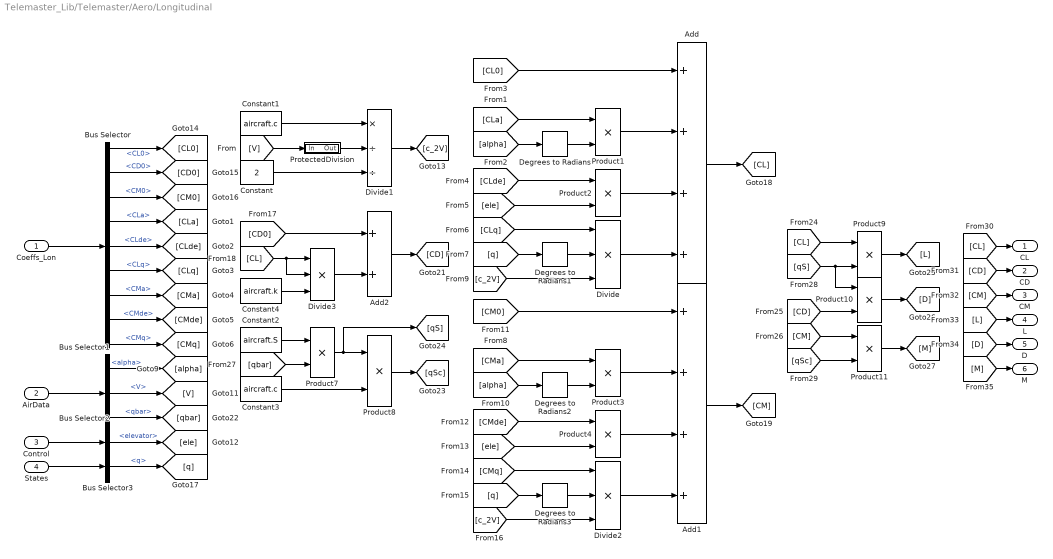
== system Telemaster_Lib/Telemaster/Aero/Longitudinal ==
  Coeffs_Lon : Inport
  AirData : Inport  Port=2
  Control : Inport  Port=3
  States : Inport  Port=4
  Add : Sum  Inputs=4
  Add1 : Sum  Inputs=4
  Add2 : Sum  Inputs=2
  Bus Selector : BusSelector  OutputSignals=CL0,CD0,CM0,CLa,CLde,CLq,CMa,CMde,CMq
  Bus Selector1 : BusSelector  OutputSignals=alpha,V,qbar
  Bus Selector2 : BusSelector  OutputSignals=elevator
  Bus Selector3 : BusSelector  OutputSignals=q
  Constant : Constant  Value=2  SampleTime=-1
  Constant1 : Constant  Value=aircraft.c  SampleTime=-1
  Constant2 : Constant  Value=aircraft.S
  Constant3 : Constant  Value=aircraft.c
  Constant4 : Constant  Value=aircraft.k
  Degrees to Radians{,1..3} (4 alike) : simulink_extras/Transformations/Degrees to Radians
  Divide : Product  Inputs=***
  Divide1 : Product  Inputs=*//
  Divide2 : Product  Inputs=***
  Divide3 : Product  Inputs=***
  Product{1..4,7..11} (9 alike) : Product
  ProtectedDivision : Subsystem
  CL : Outport
  CD : Outport  Port=2
  CM : Outport  Port=3
  L : Outport  Port=4
  D : Outport  Port=5
  M : Outport  Port=6
  wires:
  Divide3/1 -> Add2/2
  Constant4/1 -> Divide3/3
  [CL] -> Divide3/1, Divide3/2
  ProtectedDivision/1(Out) -> Divide1/2
  [L] -> L/1
  [CM] -> CM/1
  [D] -> D/1
  [CD] -> CD/1
  [M] -> M/1
  [CL] -> CL/1
  Product11/1 -> [M]
  [qSc] -> Product11/2
  [CM] -> Product11/1
  Product10/1 -> [D]
  Product9/1 -> [L]
  [CD] -> Product10/2
  [qS] -> Product9/2, Product10/1
  [CL] -> Product9/1
  Product8/1 -> [qSc]
  Constant3/1 -> Product8/2
  Product7/1 -> Product8/1, [qS]
  [qbar] -> Product7/2
  Constant2/1 -> Product7/1
  Bus Selector1/3 -> [qbar]  "<qbar>"
  Add2/1 -> [CD]
  [CD0] -> Add2/1
  [CMa] -> Product3/1
  [alpha] -> Degrees to Radians2/1
  [CMde] -> Product4/1
  [ele] -> Product4/2
  Degrees to Radians2/1 -> Product3/2
  [q] -> Degrees to Radians3/1
  Degrees to Radians3/1 -> Divide2/2
  [CMq] -> Divide2/1
  [c_2V] -> Divide2/3
  Divide2/1 -> Add1/4
  Product4/1 -> Add1/3
  Product3/1 -> Add1/2
  [CM0] -> Add1/1
  Add1/1 -> [CM]
  Add/1 -> [CL]
  [CL0] -> Add/1
  Product1/1 -> Add/2
  Product2/1 -> Add/3
  Divide/1 -> Add/4
  [c_2V] -> Divide/3
  [CLq] -> Divide/1
  Degrees to Radians1/1 -> Divide/2
  Constant1/1 -> Divide1/1
  [q] -> Degrees to Radians1/1
  Bus Selector3/1 -> [q]  "<q>"
  States/1 -> Bus Selector3/1
  Degrees to Radians/1 -> Product1/2
  [ele] -> Product2/2
  [CLde] -> Product2/1
  Bus Selector/3 -> [CM0]  "<CM0>"
  Bus Selector/2 -> [CD0]  "<CD0>"
  Bus Selector/1 -> [CL0]  "<CL0>"
  [alpha] -> Degrees to Radians/1
  [CLa] -> Product1/1
  Divide1/1 -> [c_2V]
  Constant/1 -> Divide1/3
  [V] -> ProtectedDivision/1(In)
  Bus Selector2/1 -> [ele]  "<elevator>"
  Bus Selector1/2 -> [V]  "<V>"
  Control/1 -> Bus Selector2/1
  Bus Selector1/1 -> [alpha]  "<alpha>"
  AirData/1 -> Bus Selector1/1
  Coeffs_Lon/1 -> Bus Selector/1
  Bus Selector/7 -> [CMa]  "<CMa>"
  Bus Selector/6 -> [CLq]  "<CLq>"
  Bus Selector/8 -> [CMde]  "<CMde>"
  Bus Selector/5 -> [CLde]  "<CLde>"
  Bus Selector/9 -> [CMq]  "<CMq>"
  Bus Selector/4 -> [CLa]  "<CLa>"

== system Telemaster_Lib/Telemaster/LoadFactor/ProtectedDivision ==
  In : Inport
  Compare To Zero : simulink/Logic and Bit Operations/Compare To Zero  relop===  OutDataTypeStr=boolean
  Constant : Constant  Value=1e-9  SampleTime=dt
  Switch : Switch  Criteria=u2 > Threshold  SaturateOnIntegerOverflow=off  InputSameDT=off
  Out : Outport
  wires:
  Switch/1 -> Out/1
  Compare To Zero/1 -> Switch/2
  In/1 -> Compare To Zero/1, Switch/3
  Constant/1 -> Switch/1

== system Telemaster_Lib/Telemaster/Aero/LateralDirecional/ProtectedDivision ==
  In : Inport
  Compare To Zero : simulink/Logic and Bit Operations/Compare To Zero  relop===  OutDataTypeStr=boolean
  Constant : Constant  Value=1e-9  SampleTime=-1
  Switch : Switch  Criteria=u2 > Threshold  SaturateOnIntegerOverflow=off  InputSameDT=off
  Out : Outport
  wires:
  Switch/1 -> Out/1
  Compare To Zero/1 -> Switch/2
  In/1 -> Compare To Zero/1, Switch/3
  Constant/1 -> Switch/1

== system Telemaster_Lib/Telemaster/Aero/Longitudinal/ProtectedDivision ==
  In : Inport
  Compare To Zero : simulink/Logic and Bit Operations/Compare To Zero  relop===  OutDataTypeStr=boolean
  Constant : Constant  Value=1e-9  SampleTime=-1
  Switch : Switch  Criteria=u2 > Threshold  SaturateOnIntegerOverflow=off  InputSameDT=off
  Out : Outport
  wires:
  Switch/1 -> Out/1
  Compare To Zero/1 -> Switch/2
  In/1 -> Compare To Zero/1, Switch/3
  Constant/1 -> Switch/1
